simulink model "Pokus03_Counter"  (Simulink 8.7)
settings: Solver=VariableStepAuto  StartTime=0.0  StopTime=inf  RelTol=1e-3
libraries: Bit_Multiplexers_Lib x23, simulink_extras x9, commutil2 x2
settings Model: Creator=Jozko Mrkvicka  LastModifiedBy=Jozko Mrkvicka
settings DataIOCC: LimitDataPoints=off  SaveFormat=Dataset
settings DebuggingCC: UnderspecifiedInitializationDetection=Simplified  MergeDetectMultiDrivingBlocksExec=error
settings HardwareCC: ProdBitPerPointer=64  ProdLargestAtomicFloat=Float  ProdIntDivRoundTo=Zero  ProdEndianess=LittleEndian  ProdWordSize=64  ProdHWDeviceType=Intel->x86-64 (Windows64)
settings ModelReferenceCC: PropagateSignalLabelsOutOfModel=on
settings ConfigComp: CovModelRefEnable=off

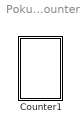
== system Pokus03_Counter ==
  Counter1 : Subsystem

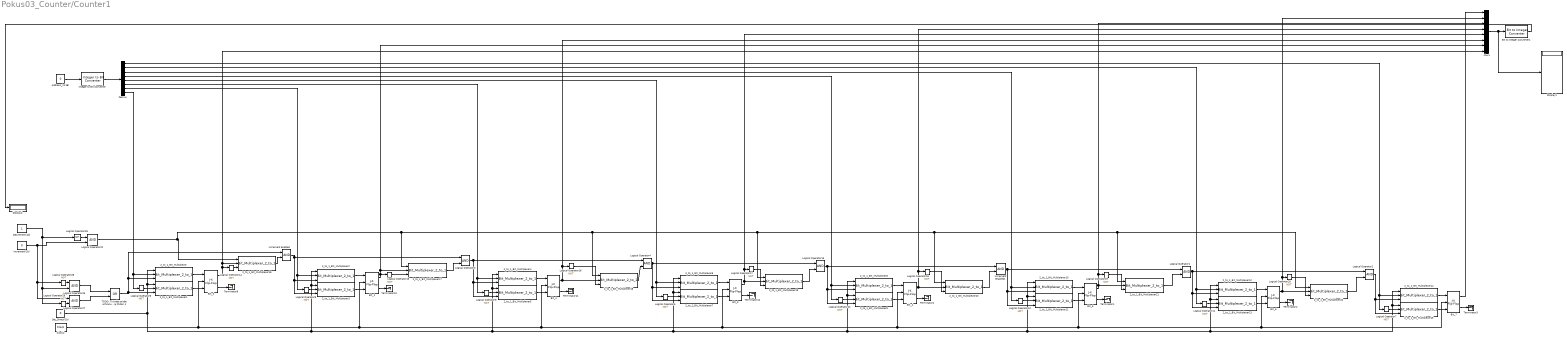
== system Pokus03_Counter/Counter1 ==
  2_to_1_Bit_Multiplexer{,1..22} (23 alike) : Bit_Multiplexers_Lib/Bit_Multiplexers_Lib/Bit_Multiplexer_2_to_1
  Address_In(1B) : Constant  Value=0  OutDataTypeStr=uint8
  Bit to Integer Converter1 : commutil2/Bit to Integer Converter  nbits=8  bitOrder=MSB first  signedOutputValues=Unsigned  outDtype=uint8  outDtypeSigned=Inherit via internal rule
  Bit_0 : simulink_extras/Flip Flops/J-K Flip-Flop  initial_condition=1
  Bit_1 : simulink_extras/Flip Flops/J-K Flip-Flop  initial_condition=1
  Bit_2 : simulink_extras/Flip Flops/J-K Flip-Flop  initial_condition=1
  Bit_{3..7} (5 alike) : simulink_extras/Flip Flops/J-K Flip-Flop  initial_condition=0
  Clock2 : simulink_extras/Flip Flops/Clock  period=1
  Decrement(1b) : Constant  OutDataTypeStr=boolean
  Demux : Demux  Outputs=8
  Display1 : Display
  Display2 : Display
  Increment Enabled : Logic  IconShape=distinctive  AllPortsSameDT=off  OutDataTypeStr=boolean
  Increment Enabled1 : Logic  IconShape=distinctive  AllPortsSameDT=off  OutDataTypeStr=boolean
  Increment(1b) : Constant  Value=0  OutDataTypeStr=boolean
  Integer to Bit Converter : commutil2/Integer to Bit Converter  nbits=8  signedInputValues=Unsigned  bitOrder=MSB first  outDtype=boolean
  Logical Operator{1..4,13,22,25,27} (8 alike) : Logic  IconShape=distinctive  AllPortsSameDT=off  OutDataTypeStr=boolean
  Logical Operator{5..12,14..20,26,28..29} (18 alike) : Logic  Operator=NOT  IconShape=distinctive  AllPortsSameDT=off  OutDataTypeStr=boolean
  Mux1 : Mux  Inputs=8
  Set_Direct(1b) : Constant  Value=0  OutDataTypeStr=boolean
  TODO: Tu treba pridat ochranu  proti stavu ked  pridu dve jednotky  (naraz instrukcia POP aj PUSH).1 : Logic  Operator=OR  IconShape=distinctive  AllPortsSameDT=off  OutDataTypeStr=boolean
  Terminator{1..4,9..12} (8 alike) : Terminator
  wires:
  2_to_1_Bit_Multiplexer18/1 -> Logical Operator4/2
  Mux1/1 -> Display1/1, Bit to Integer Converter1/1
  TODO: Tu treba pridat ochranu  proti stavu ked  pridu dve jednotky  (naraz instrukcia POP aj PUSH).1/1 -> Increment Enabled/1, 2_to_1_Bit_Multiplexer/3, 2_to_1_Bit_Multiplexer1/3
  Logical Operator3/1 -> Logical Operator4/1, 2_to_1_Bit_Multiplexer4/3, 2_to_1_Bit_Multiplexer5/3
  Logical Operator14/1 -> 2_to_1_Bit_Multiplexer16/3
  2_to_1_Bit_Multiplexer16/1 -> Increment Enabled/2
  Bit to Integer Converter1/1 -> Display2/1
  2_to_1_Bit_Multiplexer3/1 -> Bit_1/3
  Bit_0/2 -> Terminator9/1
  Logical Operator17/1 -> 2_to_1_Bit_Multiplexer19/3
  2_to_1_Bit_Multiplexer19/1 -> Logical Operator13/2
  Logical Operator19/1 -> 2_to_1_Bit_Multiplexer21/3
  2_to_1_Bit_Multiplexer/1 -> Bit_0/1
  Bit_3/1 -> 2_to_1_Bit_Multiplexer19/2, Logical Operator17/1, Mux1/5
  Logical Operator15/1 -> 2_to_1_Bit_Multiplexer17/3
  Logical Operator8/1 -> 2_to_1_Bit_Multiplexer3/2
  Bit_2/2 -> Terminator11/1
  Address_In(1B)/1 -> Integer to Bit Converter/1
  Logical Operator6/1 -> 2_to_1_Bit_Multiplexer1/2
  Bit_3/2 -> Terminator12/1
  Bit_1/1 -> 2_to_1_Bit_Multiplexer17/2, Mux1/7, Logical Operator15/1
  Bit_1/2 -> Terminator10/1
  Logical Operator18/1 -> 2_to_1_Bit_Multiplexer20/3
  Increment Enabled/1 -> 2_to_1_Bit_Multiplexer3/3, 2_to_1_Bit_Multiplexer2/3, Logical Operator3/1
  Logical Operator16/1 -> 2_to_1_Bit_Multiplexer18/3
  Demux/8 -> 2_to_1_Bit_Multiplexer/2, Logical Operator6/1
  Logical Operator20/1 -> 2_to_1_Bit_Multiplexer22/3
  Logical Operator26/1 -> Logical Operator22/1
  Bit_2/1 -> Mux1/6, Logical Operator16/1, 2_to_1_Bit_Multiplexer18/2
  2_to_1_Bit_Multiplexer2/1 -> Bit_1/1
  2_to_1_Bit_Multiplexer1/1 -> Bit_0/3
  2_to_1_Bit_Multiplexer17/1 -> Logical Operator3/2
  Logical Operator25/1 -> TODO: Tu treba pridat ochranu  proti stavu ked  pridu dve jednotky  (naraz instrukcia POP aj PUSH).1/1
  Logical Operator28/1 -> Logical Operator25/1
  Decrement(1b)/1 -> Logical Operator29/1, Logical Operator25/2, Logical Operator26/1
  Increment(1b)/1 -> Logical Operator22/2, Logical Operator27/1, Logical Operator28/1
  Logical Operator27/1 -> TODO: Tu treba pridat ochranu  proti stavu ked  pridu dve jednotky  (naraz instrukcia POP aj PUSH).1/2
  Logical Operator29/1 -> Logical Operator27/2
  2_to_1_Bit_Multiplexer22/1 -> Logical Operator2/2
  2_to_1_Bit_Multiplexer20/1 -> Increment Enabled1/2
  2_to_1_Bit_Multiplexer21/1 -> Logical Operator1/2
  Logical Operator22/1 -> 2_to_1_Bit_Multiplexer17/1, 2_to_1_Bit_Multiplexer20/1, 2_to_1_Bit_Multiplexer22/1, 2_to_1_Bit_Multiplexer21/1, 2_to_1_Bit_Multiplexer19/1, 2_to_1_Bit_Multiplexer18/1, 2_to_1_Bit_Multiplexer16/1
  2_to_1_Bit_Multiplexer15/1 -> Bit_7/3
  2_to_1_Bit_Multiplexer14/1 -> Bit_7/1
  Bit_4/1 -> 2_to_1_Bit_Multiplexer20/2, Logical Operator18/1, Mux1/4
  Demux/4 -> 2_to_1_Bit_Multiplexer8/2, Logical Operator12/1
  Logical Operator12/1 -> 2_to_1_Bit_Multiplexer9/2
  Demux/1 -> 2_to_1_Bit_Multiplexer14/2, Logical Operator7/1
  Logical Operator7/1 -> 2_to_1_Bit_Multiplexer15/2
  Logical Operator13/1 -> Increment Enabled1/1, 2_to_1_Bit_Multiplexer8/3, 2_to_1_Bit_Multiplexer9/3
  Logical Operator11/1 -> 2_to_1_Bit_Multiplexer13/2
  Demux/2 -> 2_to_1_Bit_Multiplexer12/2, Logical Operator11/1
  Clock2/1 -> Bit_7/2, Bit_6/2, Bit_5/2, Bit_4/2, Bit_3/2, Bit_2/2, Bit_1/2, Bit_0/2
  2_to_1_Bit_Multiplexer10/1 -> Bit_5/1
  Bit_7/1 -> Mux1/1
  Increment Enabled1/1 -> Logical Operator1/1, 2_to_1_Bit_Multiplexer10/3, 2_to_1_Bit_Multiplexer11/3
  Bit_6/2 -> Terminator2/1
  Set_Direct(1b)/1 -> 2_to_1_Bit_Multiplexer2/1, 2_to_1_Bit_Multiplexer3/1, 2_to_1_Bit_Multiplexer5/1, 2_to_1_Bit_Multiplexer4/1, 2_to_1_Bit_Multiplexer7/1, 2_to_1_Bit_Multiplexer6/1, 2_to_1_Bit_Multiplexer9/1, 2_to_1_Bit_Multiplexer8/1, 2_to_1_Bit_Multiplexer11/1, 2_to_1_Bit_Multiplexer10/1, 2_to_1_Bit_Multiplexer15/1, 2_to_1_Bit_Multiplexer14/1, 2_to_1_Bit_Multiplexer13/1, 2_to_1_Bit_Multiplexer12/1, 2_to_1_Bit_Multiplexer1/1, 2_to_1_Bit_Multiplexer/1
  Bit_5/2 -> Terminator1/1
  Demux/3 -> 2_to_1_Bit_Multiplexer10/2, Logical Operator10/1
  Logical Operator2/1 -> 2_to_1_Bit_Multiplexer14/3, 2_to_1_Bit_Multiplexer15/3
  2_to_1_Bit_Multiplexer11/1 -> Bit_5/3
  Bit_7/2 -> Terminator3/1
  Logical Operator1/1 -> Logical Operator2/1, 2_to_1_Bit_Multiplexer12/3, 2_to_1_Bit_Multiplexer13/3
  Bit_6/1 -> 2_to_1_Bit_Multiplexer22/2, Logical Operator20/1, Mux1/2
  2_to_1_Bit_Multiplexer9/1 -> Bit_4/3
  2_to_1_Bit_Multiplexer13/1 -> Bit_6/3
  Bit_5/1 -> Logical Operator19/1, Mux1/3, 2_to_1_Bit_Multiplexer21/2
  2_to_1_Bit_Multiplexer12/1 -> Bit_6/1
  2_to_1_Bit_Multiplexer8/1 -> Bit_4/1
  Logical Operator10/1 -> 2_to_1_Bit_Multiplexer11/2
  2_to_1_Bit_Multiplexer4/1 -> Bit_2/1
  2_to_1_Bit_Multiplexer7/1 -> Bit_3/3
  Integer to Bit Converter/1 -> Demux/1
  Logical Operator5/1 -> 2_to_1_Bit_Multiplexer7/2
  Demux/7 -> 2_to_1_Bit_Multiplexer2/2, Logical Operator8/1
  Demux/5 -> Logical Operator5/1, 2_to_1_Bit_Multiplexer6/2
  Bit_4/2 -> Terminator4/1
  2_to_1_Bit_Multiplexer6/1 -> Bit_3/1
  Logical Operator4/1 -> 2_to_1_Bit_Multiplexer7/3, 2_to_1_Bit_Multiplexer6/3, Logical Operator13/1
  Demux/6 -> 2_to_1_Bit_Multiplexer4/2, Logical Operator9/1
  Bit_0/1 -> Mux1/8, 2_to_1_Bit_Multiplexer16/2, Logical Operator14/1
  Logical Operator9/1 -> 2_to_1_Bit_Multiplexer5/2
  2_to_1_Bit_Multiplexer5/1 -> Bit_2/3
